simulink model "TP (2)"  (R2014b)
settings: Solver=ode45  StartTime=0.0  StopTime=10.0  RelTol=1e-3
values from neighbouring files (symbols this model uses):
  k = ti*0.3375    (= 1.35)    [CPI.m]    (also in Untitled.m = 1; lines.m = 6.75; tp (2).m = 1; tp.m = 1.48148148148)
  ti = 4    [CPI.m]    (also in Untitled.m = 1; lines.m = 20; tp (2).m = 2.963; tp.m = 0.5)
undefined symbols (not defined in the file or in its folder): fuite
settings Model: Creator=m1eea_002  LastModifiedBy=Bruno
settings OptimizationCC: ExpressionDepthLimit=2147483647
settings DebuggingCC: UnderspecifiedInitializationDetection=Classic  MergeDetectMultiDrivingBlocksExec=none  StateNameClashWarn=warning

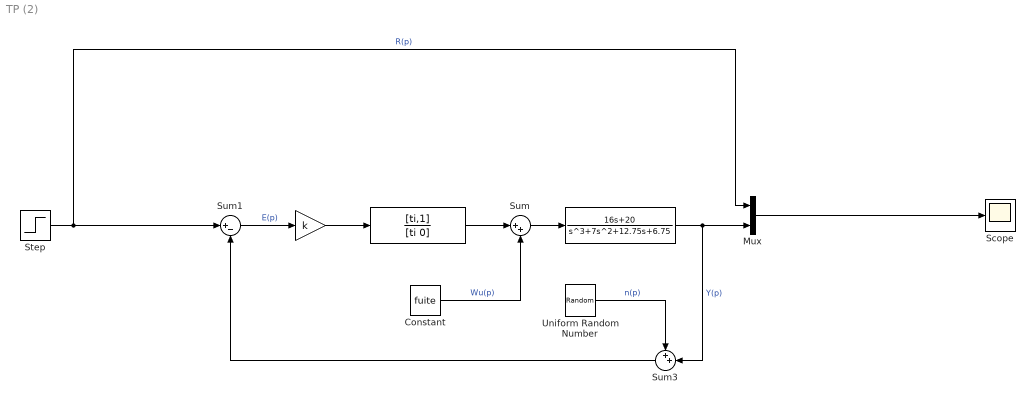
== system TP (2) ==
  " " : Gain  Gain=k
  "  " : TransferFcn  Numerator=[16,20]  Denominator=[1,7,12.75,6.75]
  "      " : TransferFcn  Numerator=[ti,1]  Denominator=[ti 0]
  Constant : Constant  Value=fuite
  Mux : Mux  Inputs=2
  Scope : Scope
  Step : Step  SampleTime=0
  Sum : Sum  Inputs=|++
  Sum1 : Sum  Inputs=|+-
  Sum3 : Sum  Inputs=++|
  Uniform Random Number : UniformRandomNumber  SampleTime=0.1
  wires:
  "  "/1 -> Sum3/2, Mux/2  "Y(p)"
  Sum/1 -> "  "/1
  "      "/1 -> Sum/1
  Step/1 -> Sum1/1, Mux/1  "R(p)"
  Mux/1 -> Scope/1
  Sum1/1 -> " "/1  "E(p)"
  " "/1 -> "      "/1
  Uniform Random Number/1 -> Sum3/1  "n(p)"
  Sum3/1 -> Sum1/2
  Constant/1 -> Sum/2  "Wu(p)"
